simulink subsystem "AC_bypass_pipe_R2024a"  (R2024a)
settings: Solver=VariableStepAuto  StartTime=0.0  StopTime=10.0  RelTol=1e-3
undefined symbols (not defined in the file or in its folder): AC_bypass_line_port_inner_area, AC_bypass_pipe_length, Ambient_temp, Initial_temp, thermal_mass_per_length_bypass, wall_thickness
libraries: fl_lib x5, nesl_utility x1
settings Model: Creator=MW  LastModifiedBy=MW

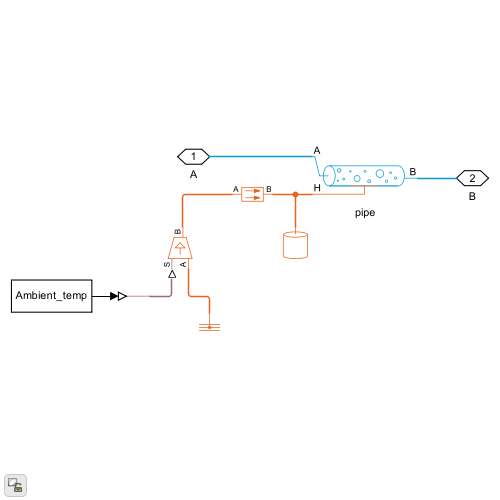
[thumbnail: Simulink's stored preview of the top-level diagram]
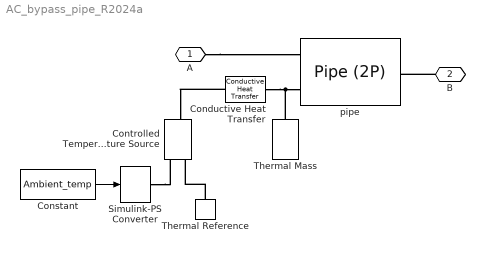
== system AC_bypass_pipe_R2024a ==
  Conductive Heat Transfer : fl_lib/Thermal/Thermal Elements/Conductive Heat Transfer  thermal_type=foundation.enum.ConstantVariableTabulated.Constant  wall_geometry=foundation.enum.ConductionWallGeometry.Cylindrical  area=hose_length m^2  thickness=0.01 m  d_in=AC_bypass_line_port_inner_area m  d_out=wall_thickness*2 + AC_bypass_line_port_inner_area m  L=AC_bypass_pipe_length m  th_cond_min=10 W/(K*m)  th_cond=pipe_thermal_conductivity W/(m*K)  th_cond_TLU=[413, 401, 392, 383, 371, 357, 342] W/(K*m)  temp_TLU=[200, 273, 400, 600, 800, 1000, 1200] K  T_specify=off  T_priority=None  T=0 K  T_nominal_specify=off  T_nominal_value=1  T_nominal_unit=K  Q_specify=off  Q_priority=None  Q=0 W  Q_nominal_specify=off  Q_nominal_value=1  Q_nominal_unit=W
  Constant : Constant  Value=Ambient_temp
  Controlled Temperature Source : fl_lib/Thermal/Thermal Sources/Controlled Temperature Source
  Simulink-PS Converter : nesl_utility/Simulink-PS Converter  PhysicalDomain=network_engine_domain  SubClassName=ps_input  LeftPortType=input  RightPortType=output  PseudoPeriodic=off  Frequencies=[]  NoiseDistribution=none  NoiseParameters=[]  Unit=1  AffineConversion=off  FilteringAndDerivatives=zero  SimscapeFilterOrder=1  InputFilterTimeConstant=0.001  UdotUserProvided=1
  Thermal Mass : fl_lib/Thermal/Thermal Elements/Thermal Mass  mass_type=foundation.enum.constant_variable.constant  mass=thermal_mass_per_length_bypass*AC_bypass_pipe_length kg  sp_heat=steel_heat_capacity J/kg/K  mass_min=1e-6 kg  num_ports=foundation.enum.numPorts2.one  m_specify=off  m_priority=High  m=1 kg  m_nominal_specify=off  m_nominal_value=1  m_nominal_unit=kg  T_specify=on  T_priority=High  T=Initial_temp K  T_nominal_specify=off  T_nominal_value=1  T_nominal_unit=K  Q_specify=off  Q_priority=None  Q=0 W  Q_nominal_specify=off  Q_nominal_value=1  Q_nominal_unit=W
  Thermal Reference : fl_lib/Thermal/Thermal Elements/Thermal Reference
  pipe : fl_lib/Two-Phase Fluid/Elements/Pipe (2P)  length=AC_bypass_pipe_length m  area=AC_bypass_line_port_inner_area m^2  Dh=AC_bypass_line_port_inner_diameter m  length_add=0.1 m  roughness=15e-6 m  Re_lam=2000  Re_tur=4000  shape_factor=64  Nu_lam=3.66  inertia=false  energy_spec=foundation.enum.energy_spec.temperature  p_init=initial_hose_p bar  T_init=Initial_temp K  x_init=0.5  alpha_init=0.5  h_init=1500 kJ/kg  u_init=1500 kJ/kg  mdot_init=0 kg/s  time_constant=0.1 s
      settings: InternalSimscapePortConfiguration="{\"Bottom\":[],\"Left\":[{\"id\":\"A\",\"label\":\"A\",\"type\":\"foundation.two_phase_fluid.two_phase_fluid\"},{\"id\":\"H\",\"label\":\"H\",\"type\":\"foundation.thermal.thermal\"}],\"Right\":[{\"id\":\"B\",\"label\":\"B\",\"type\":\"foundation.two_phase_fluid.two_phase_fluid\"}],\"Top\":[]}"
  A : PMIOPort  Side=Left
  B : PMIOPort  Port=2  Side=Right
  wires:
  Constant/1 -> Simulink-PS Converter/1
  connections:
  Conductive Heat Transfer/RConn1 -- Thermal Mass/LConn1 -- pipe/LConn2
  B/RConn1 -- pipe/RConn1
  Thermal Reference/LConn1 -- Controlled Temperature Source/RConn2
  Simulink-PS Converter/RConn1 -- Controlled Temperature Source/RConn1
  Conductive Heat Transfer/LConn1 -- Controlled Temperature Source/LConn1
  A/RConn1 -- pipe/LConn1
